simulink model "sysgenStreamedFFT"  (Simulink 7.4)
settings: Solver=VariableStepDiscrete  StartTime=0.0  StopTime=3000  RelTol=1e-3
values from neighbouring files (symbols this model uses):
  blue = blue(1:(min_x*min_y))    [makematrix.m]    (also in rgb.mat = [0 0 0 255 255 255 255 255 255 0 0 0 ... (256 elements, 256x)
  c = c(:)    [cellpipe_r13.m]    (also in cordic_sincos_script.m = xSignal; get_pipestr_r13.m = cellpipe_r13(pipestr))
  comp = [zeros(70,2) [zeros(2,66); comp; zeros(2,66)] zeros(70,2)]    [sysgenDWT_StopFcn.m]
undefined symbols (not defined in the file or in its folder): gcbh, xlBlockLoadCallback, xlipgetpartsetting
libraries: xbsIndex_r4 x117, dspxfrm3 x2, xbsCopyrightNotice_r4 x1
(part 2 of 3)

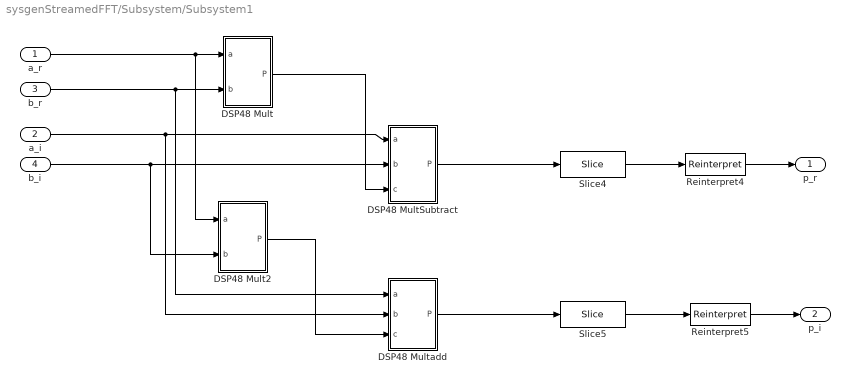
== system sysgenStreamedFFT/Subsystem/Subsystem1 ==
  a_r : Inport  OutDataType=sfix(16)  OutScaling=2^0
  a_i : Inport  Port=2  OutDataType=sfix(16)  OutScaling=2^0
  b_r : Inport  Port=3  OutDataType=sfix(16)  OutScaling=2^0
  b_i : Inport  Port=4  OutDataType=sfix(16)  OutScaling=2^0
  DSP48 Mult : Subsystem  LoadFcn=xlBlockLoadCallback(gcbh);  mask(Xilinx DSP48 Macro Block){infoedit=Macro function to simplify use of the DSP48 primitive, especially as a dynamic operator, portalist=a, portblist=b, portclist=, instrlist=|, pipeline_sgadvanced=, pipeline=Custom, pipeachoices_sgadvanced=, pipeachoices=1, pipebchoices_sgadvanced=, pipebchoices=1, pipecchoices_sgadvanced=, pipecchoices=off, pipepchoices_sgadvanced=, pipepchoices=on, pipemchoices_sgadvanced=, pipemchoices=on, pipectrlchoices_sgadvanced=, pipectrlchoices=on, pipemuxachoices_sgadvanced=, pipemuxachoices=0, pipemuxbchoices_sgadvanced=, pipemuxbchoices=0, pipemuxcchoices_sgadvanced=, pipemuxcchoices=0, pipemuxctrlchoices_sgadvanced=, pipemuxctrlchoices=0, pipeline_array_flag_sgadvanced=, pipeline_array_flag=off, custom_pipeline_cache=[1  1  0  1  1  1  0  0  0  0], precision_sgadvanced=, precision=Full, arith_type_sgadvanced=, arith_type=Signed  (2's comp), n_bits=12, bin_pt=12, bcout_sgadvanced=, bcout=off, acout_sgadvanced=, acout=off, carryout_sgadvanced=, carryout=off, carrycascout_sgadvanced=, carrycascout=off, pcout_sgadvanced=, pcout=off, rst_all_sgadvanced=, rst_all=off, rst_a_sgadvanced=, rst_a=off, rst_b_sgadvanced=, rst_b=off, rst_c_sgadvanced=, rst_c=off, rst_m_sgadvanced=, rst_m=off, rst_p_sgadvanced=, rst_p=off, rst_ctrl_sgadvanced=, rst_ctrl=off, ce_all_sgadvanced=, ce_all=off, ce_a_sgadvanced=, ce_a=off, ce_b_sgadvanced=, ce_b=off, ce_c_sgadvanced=, ce_c=off, ce_m_sgadvanced=, ce_m=off, ce_p_sgadvanced=, ce_p=off, ce_ctrl_sgadvanced=, ce_ctrl=off, dbl_ovrd_sgadvanced=, dbl_ovrd=off, synth_opt_sgadvanced=, synth_opt=on, errorlist=false, statestr=bf57e5972f25d56a71488d6ffddc6763, explicit_period=, period=1, maskdoc=, has_advanced_control=0, sggui_pos=200,234,478,593, block_type=dsp48macro, block_version=8.2.1, sg_icon_stat=45,67,2,1,white,blue,0,,right,, sg_mask_display=|, sg_list_contents=, sg_blockgui_xml=}
      mask instrlist=|
      | <html><head><meta name="qrichtext" content="1" /></head><body style="font-size:8pt;font-family:MS Shell Dlg">
      | <p>P=a*b</p>
      | </body></html>
      mask sg_mask_display=|
      | fprintf('','COMMENT: begin icon graphics');
      | patch([0 1 1 0 ],[0 0 1 1 ],[0.77 0.82 0.91]);
      | patch([0.222222 0.0666667 0.311111 0.0666667 0.222222 0.488889 0.555556 0.622222 0.911111 0.688889 0.466667 0.311111 0.555556 0.311111 0.466667 0.688889 0.911111 0.622222 0.555556 0.488889 0.222222 ],[0.238806 0.343284 0.507463 0.671642 0.776119 0.776119 0.731343 0.776119 0.776119 0.626866 0.776119 0.671642 0.507463 0.343284 0.238806 0.38806 0.238806 0.238806 0.283582 0.238806 0.238806 ],[0.98 0.96 0.92]);
      | plot([0 1 1 0 0 ],[0 0 1 1 0 ]);
      | fprintf('','COMMENT: end icon graphics');
      | fprintf('','COMMENT: begin icon text');
      | color('black');port_label('input',1,'a');
      | color('black');port_label('input',2,'b');
      | color('black');port_label('output',1,'P');
      | fprintf('','COMMENT: end icon text');
      mask prompts: infoedit ""; portalist "Inputs to port <tt>A</tt>"; portblist "Inputs to port <tt>B</tt>"; portclist "Inputs to port <tt>C</tt>"; instrlist "Instructions"; pipeline_sgadvanced ""; pipeline "Pipeline options"; pipeachoices_sgadvanced ""; pipeachoices "<tt>A</tt>"; pipebchoices_sgadvanced ""; pipebchoices "<tt>B</tt>"; pipecchoices_sgadvanced ""; pipecchoices "<tt>C</tt>"; pipepchoices_sgadvanced ""; pipepchoices "<tt>P</tt>"; pipemchoices_sgadvanced ""; pipemchoices "Multiplier"; pipectrlchoices_sgadvanced ""; pipectrlchoices "Controls (<tt>opmode</tt>, <tt>subtract</tt>,<br> <tt>carry_in</tt>, <tt>carry_in_sel</tt>)"; pipemuxachoices_sgadvanced ""; pipemuxachoices "MuxA"; pipemuxbchoices_sgadvanced ""; pipemuxbchoices "MuxB"; pipemuxcchoices_sgadvanced ""; pipemuxcchoices "MuxC"; pipemuxctrlchoices_sgadvanced ""; pipemuxctrlchoices "MuxCtrl"; pipeline_array_flag_sgadvanced ""; pipeline_array_flag "Define Using Array"; custom_pipeline_cache "Custom Pipeline Options([A,B,C,P,Ctrl,M,MuxA,MuxB,MuxC,MuxCtrl])"; precision_sgadvanced ""; arith_type_sgadvanced ""; arith_type "Output type"; n_bits "Number of bits"; bin_pt "Binary point"; bcout_sgadvanced ""; bcout "<tt>BCOUT</tt>"; acout_sgadvanced ""; acout "<tt>ACOUT</tt>"; carryout_sgadvanced ""; carryout "<tt>CARRYOUT</tt>"; carrycascout_sgadvanced ""; carrycascout "<tt>CARRYCASCOUT</tt>"; pcout_sgadvanced ""; pcout "<tt>PCOUT</tt>"; rst_all_sgadvanced ""; rst_all "<tt>Global Reset</tt>"; rst_a_sgadvanced ""; rst_a "Reset port for <tt>A</tt>"; rst_b_sgadvanced ""; rst_b "Reset port for <tt>B</tt>"; rst_c_sgadvanced ""; rst_c "Reset port for <tt>C</tt>"; rst_m_sgadvanced ""; rst_m "Reset port for multiplier"; rst_p_sgadvanced ""; rst_p "Reset port for <tt>P</tt>"; rst_ctrl_sgadvanced ""; rst_ctrl "Reset port for controls <br> (<tt>opmode</tt>, <tt>subtract</tt>,<br> <tt>carry_in</tt>, <tt>carry_in_sel</tt>)"; ce_all_sgadvanced ""; ce_all "<tt>Global Enable</tt>"; ce_a_sgadvanced ""; ce_a "Enable port for <tt>A</tt>"; ce_b_sgadvanced ""; ce_b "Enable port for <tt>B</tt>"; ce_c_sgadvanced ""; ce_c "Enable port for <tt>C</tt>"; ce_m_sgadvanced ""; ce_m "Enable port for multiplier"; ce_p_sgadvanced ""; ce_p "Enable port for <tt>P</tt>"; ce_ctrl_sgadvanced ""; ce_ctrl "Enable port for controls <br> (<tt>opmode</tt>, <tt>subtract</tt>,<br> <tt>carry_in</tt>, <tt>carry_in_sel</tt>)"; dbl_ovrd_sgadvanced ""; dbl_ovrd "Override with doubles"; synth_opt_sgadvanced ""; synth_opt "Use DSP48"; errorlist ""; statestr ""; explicit_period ""; period ""; maskdoc ""; has_advanced_control ""; sggui_pos ""; block_type ""; block_version ""; sg_icon_stat ""; sg_mask_display ""; sg_list_contents ""; sg_blockgui_xml ""
      mask help: Macro function to simplify use of the DSP48 primitive, especially as a dynamic operator
      mask init:
      | try
      |   tmp_gcb = gcb;
      |   tmp_gcbh = gcbh;
      |   xlMungeMaskParams;
      |   serialized_declarations = '{}';
      |   xldsp48macro_init();
      |   ptable_ = xlblockprep(get_param(tmp_gcb, 'MaskWSVariables'));
      | catch
      |   global dbgsysgen;
      |   if(~isempty(dbgsysgen) && dbgsysgen)
      |     e = regexprep(lasterr, '\n', '\nError: ');
      |     disp(['Error: While running MaskInit code on block ' tmp_gcb ': ' e]);
      |     error(e);
      |   end
      | end
      settings: CopyFcn=tmp_gcbh = gcbh;set_param(tmp_gcbh,'linkstatus','none');xlBlockMoveCallback(gcbh);  DeleteFcn=xlDestroyGui(gcbh);  ModelCloseFcn=xlDestroyGui(gcbh);  PreSaveFcn=xlBlockPreSaveCallback(gcbh);  PostSaveFcn=xlBlockPostSaveCallback(gcbh);  DestroyFcn=xlDestroyGui(gcbh);  OpenFcn=xlOpenGui(gcbh, 'dsp48macro_gui.xml', @dsp48macroenablement, @dsp48macroaction)  CloseFcn=xlDestroyGui(gcbh);  MoveFcn=xlBlockMoveCallback(gcbh);
      mask Help: xlWeb(xlhtmldoclink('DSP48 Macro'));
      mask StyleString: edit,edit,edit,edit,edit,edit,popup(External Registers|No External Registers|Custom),edit,popup(0|1|2),edit,popup(0|1|2),edit,checkbox,edit,checkbox,edit,checkbox,edit,checkbox,edit,popup(0|1|2),edit,popup(0|1|2),edit,popup(0|1|2),edit,popup(0|1|2),edit,checkbox,edit,edit,popup(Full|User Defined),edit,popup(Signed  (2's comp)|Unsigned),edit,edit,edit,checkbox,edit,checkbox,edit,checkbox,edit,checkbox,edit,checkbox,edit,checkbox,edit,checkbox,edit,checkbox,edit,checkbox,edit,checkbox,edit,checkbox,edit,checkbox,edit,checkbox,edit,checkbox,edit,checkbox,edit,checkbox,edit,checkbox,edit,checkbox,edit,checkbox,edit,checkbox,edit,checkbox,edit,edit,edit,edit,edit,edit,edit,edit,edit,edit,edit,edit,edit
      mask Display:
      | fprintf('','COMMENT: begin icon graphics');
      | patch([0 1 1 0 ],[0 0 1 1 ],[0.77 0.82 0.91]);
      | patch([0.222222 0.0666667 0.311111 0.0666667 0.222222 0.488889 0.555556 0.622222 0.911111 0.688889 0.466667 0.311111 0.555556 0.311111 0.466667 0.688889 0.911111 0.622222 0.555556 0.488889 0.222222 ],[0.238806 0.343284 0.507463 0.671642 0.776119 0.776119 0.731343 0.776119 0.776119 0.626866 0.776119 0.671642 0.507463 0.343284 0.238806 0.38806 0.238806 0.238806 0.283582 0.238806 0.238806 ],[0.98 0.96 0.92]);
      | plot([0 1 1 0 0 ],[0 0 1 1 0 ]);
      | fprintf('','COMMENT: end icon graphics');
      | fprintf('','COMMENT: begin icon text');
      | color('black');port_label('input',1,'a');
      | color('black');port_label('input',2,'b');
      | color('black');port_label('output',1,'P');
      | fprintf('','COMMENT: end icon text');
  DSP48 Mult2 : Subsystem  LoadFcn=xlBlockLoadCallback(gcbh);  mask(Xilinx DSP48 Macro Block){infoedit=Macro function to simplify use of the DSP48 primitive, especially as a dynamic operator, portalist=a, portblist=b, portclist=, instrlist=|, pipeline_sgadvanced=, pipeline=Custom, pipeachoices_sgadvanced=, pipeachoices=1, pipebchoices_sgadvanced=, pipebchoices=1, pipecchoices_sgadvanced=, pipecchoices=off, pipepchoices_sgadvanced=, pipepchoices=on, pipemchoices_sgadvanced=, pipemchoices=on, pipectrlchoices_sgadvanced=, pipectrlchoices=on, pipemuxachoices_sgadvanced=, pipemuxachoices=0, pipemuxbchoices_sgadvanced=, pipemuxbchoices=0, pipemuxcchoices_sgadvanced=, pipemuxcchoices=0, pipemuxctrlchoices_sgadvanced=, pipemuxctrlchoices=0, pipeline_array_flag_sgadvanced=, pipeline_array_flag=off, custom_pipeline_cache=[1  1  0  1  1  1  0  0  0  0], precision_sgadvanced=, precision=Full, arith_type_sgadvanced=, arith_type=Signed  (2's comp), n_bits=12, bin_pt=12, bcout_sgadvanced=, bcout=off, acout_sgadvanced=, acout=off, carryout_sgadvanced=, carryout=off, carrycascout_sgadvanced=, carrycascout=off, pcout_sgadvanced=, pcout=off, rst_all_sgadvanced=, rst_all=off, rst_a_sgadvanced=, rst_a=off, rst_b_sgadvanced=, rst_b=off, rst_c_sgadvanced=, rst_c=off, rst_m_sgadvanced=, rst_m=off, rst_p_sgadvanced=, rst_p=off, rst_ctrl_sgadvanced=, rst_ctrl=off, ce_all_sgadvanced=, ce_all=off, ce_a_sgadvanced=, ce_a=off, ce_b_sgadvanced=, ce_b=off, ce_c_sgadvanced=, ce_c=off, ce_m_sgadvanced=, ce_m=off, ce_p_sgadvanced=, ce_p=off, ce_ctrl_sgadvanced=, ce_ctrl=off, dbl_ovrd_sgadvanced=, dbl_ovrd=off, synth_opt_sgadvanced=, synth_opt=on, errorlist=false, statestr=bf57e5972f25d56a71488d6ffddc6763, explicit_period=, period=1, maskdoc=, has_advanced_control=0, sggui_pos=429,230,426,499, block_type=dsp48macro, block_version=8.2.1, sg_icon_stat=45,67,2,1,white,blue,0,,right,, sg_mask_display=|, sg_list_contents=, sg_blockgui_xml=}
      mask instrlist=|
      | <html><head><meta name="qrichtext" content="1" /></head><body style="font-size:8pt;font-family:MS Shell Dlg">
      | <p>P=a*b</p>
      | </body></html>
      mask sg_mask_display=|
      | fprintf('','COMMENT: begin icon graphics');
      | patch([0 1 1 0 ],[0 0 1 1 ],[0.77 0.82 0.91]);
      | patch([0.222222 0.0666667 0.311111 0.0666667 0.222222 0.488889 0.555556 0.622222 0.911111 0.688889 0.466667 0.311111 0.555556 0.311111 0.466667 0.688889 0.911111 0.622222 0.555556 0.488889 0.222222 ],[0.238806 0.343284 0.507463 0.671642 0.776119 0.776119 0.731343 0.776119 0.776119 0.626866 0.776119 0.671642 0.507463 0.343284 0.238806 0.38806 0.238806 0.238806 0.283582 0.238806 0.238806 ],[0.98 0.96 0.92]);
      | plot([0 1 1 0 0 ],[0 0 1 1 0 ]);
      | fprintf('','COMMENT: end icon graphics');
      | fprintf('','COMMENT: begin icon text');
      | color('black');port_label('input',1,'a');
      | color('black');port_label('input',2,'b');
      | color('black');port_label('output',1,'P');
      | fprintf('','COMMENT: end icon text');
      mask prompts: infoedit ""; portalist "Inputs to port <tt>A</tt>"; portblist "Inputs to port <tt>B</tt>"; portclist "Inputs to port <tt>C</tt>"; instrlist "Instructions"; pipeline_sgadvanced ""; pipeline "Pipeline options"; pipeachoices_sgadvanced ""; pipeachoices "<tt>A</tt>"; pipebchoices_sgadvanced ""; pipebchoices "<tt>B</tt>"; pipecchoices_sgadvanced ""; pipecchoices "<tt>C</tt>"; pipepchoices_sgadvanced ""; pipepchoices "<tt>P</tt>"; pipemchoices_sgadvanced ""; pipemchoices "Multiplier"; pipectrlchoices_sgadvanced ""; pipectrlchoices "Controls (<tt>opmode</tt>, <tt>subtract</tt>,<br> <tt>carry_in</tt>, <tt>carry_in_sel</tt>)"; pipemuxachoices_sgadvanced ""; pipemuxachoices "MuxA"; pipemuxbchoices_sgadvanced ""; pipemuxbchoices "MuxB"; pipemuxcchoices_sgadvanced ""; pipemuxcchoices "MuxC"; pipemuxctrlchoices_sgadvanced ""; pipemuxctrlchoices "MuxCtrl"; pipeline_array_flag_sgadvanced ""; pipeline_array_flag "Define Using Array"; custom_pipeline_cache "Custom Pipeline Options([A,B,C,P,Ctrl,M,MuxA,MuxB,MuxC,MuxCtrl])"; precision_sgadvanced ""; arith_type_sgadvanced ""; arith_type "Output type"; n_bits "Number of bits"; bin_pt "Binary point"; bcout_sgadvanced ""; bcout "<tt>BCOUT</tt>"; acout_sgadvanced ""; acout "<tt>ACOUT</tt>"; carryout_sgadvanced ""; carryout "<tt>CARRYOUT</tt>"; carrycascout_sgadvanced ""; carrycascout "<tt>CARRYCASCOUT</tt>"; pcout_sgadvanced ""; pcout "<tt>PCOUT</tt>"; rst_all_sgadvanced ""; rst_all "<tt>Global Reset</tt>"; rst_a_sgadvanced ""; rst_a "Reset port for <tt>A</tt>"; rst_b_sgadvanced ""; rst_b "Reset port for <tt>B</tt>"; rst_c_sgadvanced ""; rst_c "Reset port for <tt>C</tt>"; rst_m_sgadvanced ""; rst_m "Reset port for multiplier"; rst_p_sgadvanced ""; rst_p "Reset port for <tt>P</tt>"; rst_ctrl_sgadvanced ""; rst_ctrl "Reset port for controls <br> (<tt>opmode</tt>, <tt>subtract</tt>,<br> <tt>carry_in</tt>, <tt>carry_in_sel</tt>)"; ce_all_sgadvanced ""; ce_all "<tt>Global Enable</tt>"; ce_a_sgadvanced ""; ce_a "Enable port for <tt>A</tt>"; ce_b_sgadvanced ""; ce_b "Enable port for <tt>B</tt>"; ce_c_sgadvanced ""; ce_c "Enable port for <tt>C</tt>"; ce_m_sgadvanced ""; ce_m "Enable port for multiplier"; ce_p_sgadvanced ""; ce_p "Enable port for <tt>P</tt>"; ce_ctrl_sgadvanced ""; ce_ctrl "Enable port for controls <br> (<tt>opmode</tt>, <tt>subtract</tt>,<br> <tt>carry_in</tt>, <tt>carry_in_sel</tt>)"; dbl_ovrd_sgadvanced ""; dbl_ovrd "Override with doubles"; synth_opt_sgadvanced ""; synth_opt "Use DSP48"; errorlist ""; statestr ""; explicit_period ""; period ""; maskdoc ""; has_advanced_control ""; sggui_pos ""; block_type ""; block_version ""; sg_icon_stat ""; sg_mask_display ""; sg_list_contents ""; sg_blockgui_xml ""
      mask help: Macro function to simplify use of the DSP48 primitive, especially as a dynamic operator
      mask init: same as sysgenStreamedFFT/Subsystem/Subsystem1/DSP48 Mult
      settings: CopyFcn=tmp_gcbh = gcbh;set_param(tmp_gcbh,'linkstatus','none');xlBlockMoveCallback(gcbh);  DeleteFcn=xlDestroyGui(gcbh);  ModelCloseFcn=xlDestroyGui(gcbh);  PreSaveFcn=xlBlockPreSaveCallback(gcbh);  PostSaveFcn=xlBlockPostSaveCallback(gcbh);  DestroyFcn=xlDestroyGui(gcbh);  OpenFcn=xlOpenGui(gcbh, 'dsp48macro_gui.xml', @dsp48macroenablement, @dsp48macroaction)  CloseFcn=xlDestroyGui(gcbh);  MoveFcn=xlBlockMoveCallback(gcbh);
      mask Help: xlWeb(xlhtmldoclink('DSP48 Macro'));
      mask StyleString: edit,edit,edit,edit,edit,edit,popup(External Registers|No External Registers|Custom),edit,popup(0|1|2),edit,popup(0|1|2),edit,checkbox,edit,checkbox,edit,checkbox,edit,checkbox,edit,popup(0|1|2),edit,popup(0|1|2),edit,popup(0|1|2),edit,popup(0|1|2),edit,checkbox,edit,edit,popup(Full|User Defined),edit,popup(Signed  (2's comp)|Unsigned),edit,edit,edit,checkbox,edit,checkbox,edit,checkbox,edit,checkbox,edit,checkbox,edit,checkbox,edit,checkbox,edit,checkbox,edit,checkbox,edit,checkbox,edit,checkbox,edit,checkbox,edit,checkbox,edit,checkbox,edit,checkbox,edit,checkbox,edit,checkbox,edit,checkbox,edit,checkbox,edit,checkbox,edit,checkbox,edit,edit,edit,edit,edit,edit,edit,edit,edit,edit,edit,edit,edit
      mask Display:
      | fprintf('','COMMENT: begin icon graphics');
      | patch([0 1 1 0 ],[0 0 1 1 ],[0.77 0.82 0.91]);
      | patch([0.222222 0.0666667 0.311111 0.0666667 0.222222 0.488889 0.555556 0.622222 0.911111 0.688889 0.466667 0.311111 0.555556 0.311111 0.466667 0.688889 0.911111 0.622222 0.555556 0.488889 0.222222 ],[0.238806 0.343284 0.507463 0.671642 0.776119 0.776119 0.731343 0.776119 0.776119 0.626866 0.776119 0.671642 0.507463 0.343284 0.238806 0.38806 0.238806 0.238806 0.283582 0.238806 0.238806 ],[0.98 0.96 0.92]);
      | plot([0 1 1 0 0 ],[0 0 1 1 0 ]);
      | fprintf('','COMMENT: end icon graphics');
      | fprintf('','COMMENT: begin icon text');
      | color('black');port_label('input',1,'a');
      | color('black');port_label('input',2,'b');
      | color('black');port_label('output',1,'P');
      | fprintf('','COMMENT: end icon text');
  DSP48 MultSubtract : Subsystem  LoadFcn=xlBlockLoadCallback(gcbh);  mask(Xilinx DSP48 Macro Block){infoedit=Macro function to simplify use of the DSP48 primitive, especially as a dynamic operator, portalist=a, portblist=b, portclist=c, instrlist=|, pipeline_sgadvanced=, pipeline=Custom, pipeachoices_sgadvanced=, pipeachoices=1, pipebchoices_sgadvanced=, pipebchoices=1, pipecchoices_sgadvanced=, pipecchoices=on, pipepchoices_sgadvanced=, pipepchoices=on, pipemchoices_sgadvanced=, pipemchoices=on, pipectrlchoices_sgadvanced=, pipectrlchoices=on, pipemuxachoices_sgadvanced=, pipemuxachoices=0, pipemuxbchoices_sgadvanced=, pipemuxbchoices=0, pipemuxcchoices_sgadvanced=, pipemuxcchoices=0, pipemuxctrlchoices_sgadvanced=, pipemuxctrlchoices=0, pipeline_array_flag_sgadvanced=, pipeline_array_flag=off, custom_pipeline_cache=[1  1  1  1  1  1  0  0  0  0], precision_sgadvanced=, precision=Full, arith_type_sgadvanced=, arith_type=Signed  (2's comp), n_bits=12, bin_pt=12, bcout_sgadvanced=, bcout=off, acout_sgadvanced=, acout=off, carryout_sgadvanced=, carryout=off, carrycascout_sgadvanced=, carrycascout=off, pcout_sgadvanced=, pcout=off, rst_all_sgadvanced=, rst_all=off, rst_a_sgadvanced=, rst_a=off, rst_b_sgadvanced=, rst_b=off, rst_c_sgadvanced=, rst_c=off, rst_m_sgadvanced=, rst_m=off, rst_p_sgadvanced=, rst_p=off, rst_ctrl_sgadvanced=, rst_ctrl=off, ce_all_sgadvanced=, ce_all=off, ce_a_sgadvanced=, ce_a=off, ce_b_sgadvanced=, ce_b=off, ce_c_sgadvanced=, ce_c=off, ce_m_sgadvanced=, ce_m=off, ce_p_sgadvanced=, ce_p=off, ce_ctrl_sgadvanced=, ce_ctrl=off, dbl_ovrd_sgadvanced=, dbl_ovrd=off, synth_opt_sgadvanced=, synth_opt=on, errorlist=false, statestr=e43659f44466f7be952996a9572528ef, explicit_period=, period=1, maskdoc=, has_advanced_control=0, sggui_pos=429,230,478,550, block_type=dsp48macro, block_version=8.2.1, sg_icon_stat=45,74,3,1,white,blue,0,,right,, sg_mask_display=|, sg_list_contents=, sg_blockgui_xml=}
      mask instrlist=|
      | <html><head><meta name="qrichtext" content="1" /></head><body style="font-size:8pt;font-family:MS Shell Dlg">
      | <p>P=c-a*b</p>
      | </body></html>
      mask sg_mask_display=|
      | fprintf('','COMMENT: begin icon graphics');
      | patch([0 1 1 0 ],[0 0 1 1 ],[0.77 0.82 0.91]);
      | patch([0.222222 0.0666667 0.311111 0.0666667 0.222222 0.488889 0.555556 0.622222 0.911111 0.688889 0.466667 0.311111 0.555556 0.311111 0.466667 0.688889 0.911111 0.622222 0.555556 0.488889 0.222222 ],[0.256757 0.351351 0.5 0.648649 0.743243 0.743243 0.702703 0.743243 0.743243 0.608108 0.743243 0.648649 0.5 0.351351 0.256757 0.391892 0.256757 0.256757 0.297297 0.256757 0.256757 ],[0.98 0.96 0.92]);
      | plot([0 1 1 0 0 ],[0 0 1 1 0 ]);
      | fprintf('','COMMENT: end icon graphics');
      | fprintf('','COMMENT: begin icon text');
      | color('black');port_label('input',1,'a');
      | color('black');port_label('input',2,'b');
      | color('black');port_label('input',3,'c');
      | color('black');port_label('output',1,'P');
      | fprintf('','COMMENT: end icon text');
      mask prompts: infoedit ""; portalist "Inputs to port <tt>A</tt>"; portblist "Inputs to port <tt>B</tt>"; portclist "Inputs to port <tt>C</tt>"; instrlist "Instructions"; pipeline_sgadvanced ""; pipeline "Pipeline options"; pipeachoices_sgadvanced ""; pipeachoices "<tt>A</tt>"; pipebchoices_sgadvanced ""; pipebchoices "<tt>B</tt>"; pipecchoices_sgadvanced ""; pipecchoices "<tt>C</tt>"; pipepchoices_sgadvanced ""; pipepchoices "<tt>P</tt>"; pipemchoices_sgadvanced ""; pipemchoices "Multiplier"; pipectrlchoices_sgadvanced ""; pipectrlchoices "Controls (<tt>opmode</tt>, <tt>subtract</tt>,<br> <tt>carry_in</tt>, <tt>carry_in_sel</tt>)"; pipemuxachoices_sgadvanced ""; pipemuxachoices "MuxA"; pipemuxbchoices_sgadvanced ""; pipemuxbchoices "MuxB"; pipemuxcchoices_sgadvanced ""; pipemuxcchoices "MuxC"; pipemuxctrlchoices_sgadvanced ""; pipemuxctrlchoices "MuxCtrl"; pipeline_array_flag_sgadvanced ""; pipeline_array_flag "Define Using Array"; custom_pipeline_cache "Custom Pipeline Options([A,B,C,P,Ctrl,M,MuxA,MuxB,MuxC,MuxCtrl])"; precision_sgadvanced ""; arith_type_sgadvanced ""; arith_type "Output type"; n_bits "Number of bits"; bin_pt "Binary point"; bcout_sgadvanced ""; bcout "<tt>BCOUT</tt>"; acout_sgadvanced ""; acout "<tt>ACOUT</tt>"; carryout_sgadvanced ""; carryout "<tt>CARRYOUT</tt>"; carrycascout_sgadvanced ""; carrycascout "<tt>CARRYCASCOUT</tt>"; pcout_sgadvanced ""; pcout "<tt>PCOUT</tt>"; rst_all_sgadvanced ""; rst_all "<tt>Global Reset</tt>"; rst_a_sgadvanced ""; rst_a "Reset port for <tt>A</tt>"; rst_b_sgadvanced ""; rst_b "Reset port for <tt>B</tt>"; rst_c_sgadvanced ""; rst_c "Reset port for <tt>C</tt>"; rst_m_sgadvanced ""; rst_m "Reset port for multiplier"; rst_p_sgadvanced ""; rst_p "Reset port for <tt>P</tt>"; rst_ctrl_sgadvanced ""; rst_ctrl "Reset port for controls <br> (<tt>opmode</tt>, <tt>subtract</tt>,<br> <tt>carry_in</tt>, <tt>carry_in_sel</tt>)"; ce_all_sgadvanced ""; ce_all "<tt>Global Enable</tt>"; ce_a_sgadvanced ""; ce_a "Enable port for <tt>A</tt>"; ce_b_sgadvanced ""; ce_b "Enable port for <tt>B</tt>"; ce_c_sgadvanced ""; ce_c "Enable port for <tt>C</tt>"; ce_m_sgadvanced ""; ce_m "Enable port for multiplier"; ce_p_sgadvanced ""; ce_p "Enable port for <tt>P</tt>"; ce_ctrl_sgadvanced ""; ce_ctrl "Enable port for controls <br> (<tt>opmode</tt>, <tt>subtract</tt>,<br> <tt>carry_in</tt>, <tt>carry_in_sel</tt>)"; dbl_ovrd_sgadvanced ""; dbl_ovrd "Override with doubles"; synth_opt_sgadvanced ""; synth_opt "Use DSP48"; errorlist ""; statestr ""; explicit_period ""; period ""; maskdoc ""; has_advanced_control ""; sggui_pos ""; block_type ""; block_version ""; sg_icon_stat ""; sg_mask_display ""; sg_list_contents ""; sg_blockgui_xml ""
      mask help: Macro function to simplify use of the DSP48 primitive, especially as a dynamic operator
      mask init: same as sysgenStreamedFFT/Subsystem/Subsystem1/DSP48 Mult
      settings: CopyFcn=tmp_gcbh = gcbh;set_param(tmp_gcbh,'linkstatus','none');xlBlockMoveCallback(gcbh);  DeleteFcn=xlDestroyGui(gcbh);  ModelCloseFcn=xlDestroyGui(gcbh);  PreSaveFcn=xlBlockPreSaveCallback(gcbh);  PostSaveFcn=xlBlockPostSaveCallback(gcbh);  DestroyFcn=xlDestroyGui(gcbh);  OpenFcn=xlOpenGui(gcbh, 'dsp48macro_gui.xml', @dsp48macroenablement, @dsp48macroaction)  CloseFcn=xlDestroyGui(gcbh);  MoveFcn=xlBlockMoveCallback(gcbh);
      mask Help: xlWeb(xlhtmldoclink('DSP48 Macro'));
      mask StyleString: edit,edit,edit,edit,edit,edit,popup(External Registers|No External Registers|Custom),edit,popup(0|1|2),edit,popup(0|1|2),edit,checkbox,edit,checkbox,edit,checkbox,edit,checkbox,edit,popup(0|1|2),edit,popup(0|1|2),edit,popup(0|1|2),edit,popup(0|1|2),edit,checkbox,edit,edit,popup(Full|User Defined),edit,popup(Signed  (2's comp)|Unsigned),edit,edit,edit,checkbox,edit,checkbox,edit,checkbox,edit,checkbox,edit,checkbox,edit,checkbox,edit,checkbox,edit,checkbox,edit,checkbox,edit,checkbox,edit,checkbox,edit,checkbox,edit,checkbox,edit,checkbox,edit,checkbox,edit,checkbox,edit,checkbox,edit,checkbox,edit,checkbox,edit,checkbox,edit,checkbox,edit,edit,edit,edit,edit,edit,edit,edit,edit,edit,edit,edit,edit
      mask Display:
      | fprintf('','COMMENT: begin icon graphics');
      | patch([0 1 1 0 ],[0 0 1 1 ],[0.77 0.82 0.91]);
      | patch([0.222222 0.0666667 0.311111 0.0666667 0.222222 0.488889 0.555556 0.622222 0.911111 0.688889 0.466667 0.311111 0.555556 0.311111 0.466667 0.688889 0.911111 0.622222 0.555556 0.488889 0.222222 ],[0.256757 0.351351 0.5 0.648649 0.743243 0.743243 0.702703 0.743243 0.743243 0.608108 0.743243 0.648649 0.5 0.351351 0.256757 0.391892 0.256757 0.256757 0.297297 0.256757 0.256757 ],[0.98 0.96 0.92]);
      | plot([0 1 1 0 0 ],[0 0 1 1 0 ]);
      | fprintf('','COMMENT: end icon graphics');
      | fprintf('','COMMENT: begin icon text');
      | color('black');port_label('input',1,'a');
      | color('black');port_label('input',2,'b');
      | color('black');port_label('input',3,'c');
      | color('black');port_label('output',1,'P');
      | fprintf('','COMMENT: end icon text');
  DSP48 Multadd : Subsystem  LoadFcn=xlBlockLoadCallback(gcbh);  mask(Xilinx DSP48 Macro Block){infoedit=Macro function to simplify use of the DSP48 primitive, especially as a dynamic operator, portalist=a, portblist=b, portclist=c, instrlist=|, pipeline_sgadvanced=, pipeline=Custom, pipeachoices_sgadvanced=, pipeachoices=1, pipebchoices_sgadvanced=, pipebchoices=1, pipecchoices_sgadvanced=, pipecchoices=on, pipepchoices_sgadvanced=, pipepchoices=on, pipemchoices_sgadvanced=, pipemchoices=on, pipectrlchoices_sgadvanced=, pipectrlchoices=on, pipemuxachoices_sgadvanced=, pipemuxachoices=0, pipemuxbchoices_sgadvanced=, pipemuxbchoices=0, pipemuxcchoices_sgadvanced=, pipemuxcchoices=0, pipemuxctrlchoices_sgadvanced=, pipemuxctrlchoices=0, pipeline_array_flag_sgadvanced=, pipeline_array_flag=off, custom_pipeline_cache=[1  1  1  1  1  1  0  0  0  0], precision_sgadvanced=, precision=Full, arith_type_sgadvanced=, arith_type=Signed  (2's comp), n_bits=12, bin_pt=12, bcout_sgadvanced=, bcout=off, acout_sgadvanced=, acout=off, carryout_sgadvanced=, carryout=off, carrycascout_sgadvanced=, carrycascout=off, pcout_sgadvanced=, pcout=off, rst_all_sgadvanced=, rst_all=off, rst_a_sgadvanced=, rst_a=off, rst_b_sgadvanced=, rst_b=off, rst_c_sgadvanced=, rst_c=off, rst_m_sgadvanced=, rst_m=off, rst_p_sgadvanced=, rst_p=off, rst_ctrl_sgadvanced=, rst_ctrl=off, ce_all_sgadvanced=, ce_all=off, ce_a_sgadvanced=, ce_a=off, ce_b_sgadvanced=, ce_b=off, ce_c_sgadvanced=, ce_c=off, ce_m_sgadvanced=, ce_m=off, ce_p_sgadvanced=, ce_p=off, ce_ctrl_sgadvanced=, ce_ctrl=off, dbl_ovrd_sgadvanced=, dbl_ovrd=off, synth_opt_sgadvanced=, synth_opt=on, errorlist=false, statestr=e63290abb6eb2d1c13234b0ccbf6f8a4, explicit_period=, period=1, maskdoc=, has_advanced_control=0, sggui_pos=429,230,426,499, block_type=dsp48macro, block_version=8.2.1, sg_icon_stat=45,68,3,1,white,blue,0,,right,, sg_mask_display=|, sg_list_contents=, sg_blockgui_xml=}
      mask instrlist=|
      | <html><head><meta name="qrichtext" content="1" /></head><body style="font-size:8pt;font-family:MS Shell Dlg">
      | <p>P=c+a*b</p>
      | </body></html>
      mask sg_mask_display=|
      | fprintf('','COMMENT: begin icon graphics');
      | patch([0 1 1 0 ],[0 0 1 1 ],[0.77 0.82 0.91]);
      | patch([0.222222 0.0666667 0.311111 0.0666667 0.222222 0.488889 0.555556 0.622222 0.911111 0.688889 0.466667 0.311111 0.555556 0.311111 0.466667 0.688889 0.911111 0.622222 0.555556 0.488889 0.222222 ],[0.235294 0.338235 0.5 0.661765 0.764706 0.764706 0.720588 0.764706 0.764706 0.617647 0.764706 0.661765 0.5 0.338235 0.235294 0.382353 0.235294 0.235294 0.279412 0.235294 0.235294 ],[0.98 0.96 0.92]);
      | plot([0 1 1 0 0 ],[0 0 1 1 0 ]);
      | fprintf('','COMMENT: end icon graphics');
      | fprintf('','COMMENT: begin icon text');
      | color('black');port_label('input',1,'a');
      | color('black');port_label('input',2,'b');
      | color('black');port_label('input',3,'c');
      | color('black');port_label('output',1,'P');
      | fprintf('','COMMENT: end icon text');
      mask prompts: infoedit ""; portalist "Inputs to port <tt>A</tt>"; portblist "Inputs to port <tt>B</tt>"; portclist "Inputs to port <tt>C</tt>"; instrlist "Instructions"; pipeline_sgadvanced ""; pipeline "Pipeline options"; pipeachoices_sgadvanced ""; pipeachoices "<tt>A</tt>"; pipebchoices_sgadvanced ""; pipebchoices "<tt>B</tt>"; pipecchoices_sgadvanced ""; pipecchoices "<tt>C</tt>"; pipepchoices_sgadvanced ""; pipepchoices "<tt>P</tt>"; pipemchoices_sgadvanced ""; pipemchoices "Multiplier"; pipectrlchoices_sgadvanced ""; pipectrlchoices "Controls (<tt>opmode</tt>, <tt>subtract</tt>,<br> <tt>carry_in</tt>, <tt>carry_in_sel</tt>)"; pipemuxachoices_sgadvanced ""; pipemuxachoices "MuxA"; pipemuxbchoices_sgadvanced ""; pipemuxbchoices "MuxB"; pipemuxcchoices_sgadvanced ""; pipemuxcchoices "MuxC"; pipemuxctrlchoices_sgadvanced ""; pipemuxctrlchoices "MuxCtrl"; pipeline_array_flag_sgadvanced ""; pipeline_array_flag "Define Using Array"; custom_pipeline_cache "Custom Pipeline Options([A,B,C,P,Ctrl,M,MuxA,MuxB,MuxC,MuxCtrl])"; precision_sgadvanced ""; arith_type_sgadvanced ""; arith_type "Output type"; n_bits "Number of bits"; bin_pt "Binary point"; bcout_sgadvanced ""; bcout "<tt>BCOUT</tt>"; acout_sgadvanced ""; acout "<tt>ACOUT</tt>"; carryout_sgadvanced ""; carryout "<tt>CARRYOUT</tt>"; carrycascout_sgadvanced ""; carrycascout "<tt>CARRYCASCOUT</tt>"; pcout_sgadvanced ""; pcout "<tt>PCOUT</tt>"; rst_all_sgadvanced ""; rst_all "<tt>Global Reset</tt>"; rst_a_sgadvanced ""; rst_a "Reset port for <tt>A</tt>"; rst_b_sgadvanced ""; rst_b "Reset port for <tt>B</tt>"; rst_c_sgadvanced ""; rst_c "Reset port for <tt>C</tt>"; rst_m_sgadvanced ""; rst_m "Reset port for multiplier"; rst_p_sgadvanced ""; rst_p "Reset port for <tt>P</tt>"; rst_ctrl_sgadvanced ""; rst_ctrl "Reset port for controls <br> (<tt>opmode</tt>, <tt>subtract</tt>,<br> <tt>carry_in</tt>, <tt>carry_in_sel</tt>)"; ce_all_sgadvanced ""; ce_all "<tt>Global Enable</tt>"; ce_a_sgadvanced ""; ce_a "Enable port for <tt>A</tt>"; ce_b_sgadvanced ""; ce_b "Enable port for <tt>B</tt>"; ce_c_sgadvanced ""; ce_c "Enable port for <tt>C</tt>"; ce_m_sgadvanced ""; ce_m "Enable port for multiplier"; ce_p_sgadvanced ""; ce_p "Enable port for <tt>P</tt>"; ce_ctrl_sgadvanced ""; ce_ctrl "Enable port for controls <br> (<tt>opmode</tt>, <tt>subtract</tt>,<br> <tt>carry_in</tt>, <tt>carry_in_sel</tt>)"; dbl_ovrd_sgadvanced ""; dbl_ovrd "Override with doubles"; synth_opt_sgadvanced ""; synth_opt "Use DSP48"; errorlist ""; statestr ""; explicit_period ""; period ""; maskdoc ""; has_advanced_control ""; sggui_pos ""; block_type ""; block_version ""; sg_icon_stat ""; sg_mask_display ""; sg_list_contents ""; sg_blockgui_xml ""
      mask help: Macro function to simplify use of the DSP48 primitive, especially as a dynamic operator
      mask init: same as sysgenStreamedFFT/Subsystem/Subsystem1/DSP48 Mult
      settings: CopyFcn=tmp_gcbh = gcbh;set_param(tmp_gcbh,'linkstatus','none');xlBlockMoveCallback(gcbh);  DeleteFcn=xlDestroyGui(gcbh);  ModelCloseFcn=xlDestroyGui(gcbh);  PreSaveFcn=xlBlockPreSaveCallback(gcbh);  PostSaveFcn=xlBlockPostSaveCallback(gcbh);  DestroyFcn=xlDestroyGui(gcbh);  OpenFcn=xlOpenGui(gcbh, 'dsp48macro_gui.xml', @dsp48macroenablement, @dsp48macroaction)  CloseFcn=xlDestroyGui(gcbh);  MoveFcn=xlBlockMoveCallback(gcbh);
      mask Help: xlWeb(xlhtmldoclink('DSP48 Macro'));
      mask StyleString: edit,edit,edit,edit,edit,edit,popup(External Registers|No External Registers|Custom),edit,popup(0|1|2),edit,popup(0|1|2),edit,checkbox,edit,checkbox,edit,checkbox,edit,checkbox,edit,popup(0|1|2),edit,popup(0|1|2),edit,popup(0|1|2),edit,popup(0|1|2),edit,checkbox,edit,edit,popup(Full|User Defined),edit,popup(Signed  (2's comp)|Unsigned),edit,edit,edit,checkbox,edit,checkbox,edit,checkbox,edit,checkbox,edit,checkbox,edit,checkbox,edit,checkbox,edit,checkbox,edit,checkbox,edit,checkbox,edit,checkbox,edit,checkbox,edit,checkbox,edit,checkbox,edit,checkbox,edit,checkbox,edit,checkbox,edit,checkbox,edit,checkbox,edit,checkbox,edit,checkbox,edit,edit,edit,edit,edit,edit,edit,edit,edit,edit,edit,edit,edit
      mask Display:
      | fprintf('','COMMENT: begin icon graphics');
      | patch([0 1 1 0 ],[0 0 1 1 ],[0.77 0.82 0.91]);
      | patch([0.222222 0.0666667 0.311111 0.0666667 0.222222 0.488889 0.555556 0.622222 0.911111 0.688889 0.466667 0.311111 0.555556 0.311111 0.466667 0.688889 0.911111 0.622222 0.555556 0.488889 0.222222 ],[0.235294 0.338235 0.5 0.661765 0.764706 0.764706 0.720588 0.764706 0.764706 0.617647 0.764706 0.661765 0.5 0.338235 0.235294 0.382353 0.235294 0.235294 0.279412 0.235294 0.235294 ],[0.98 0.96 0.92]);
      | plot([0 1 1 0 0 ],[0 0 1 1 0 ]);
      | fprintf('','COMMENT: end icon graphics');
      | fprintf('','COMMENT: begin icon text');
      | color('black');port_label('input',1,'a');
      | color('black');port_label('input',2,'b');
      | color('black');port_label('input',3,'c');
      | color('black');port_label('output',1,'P');
      | fprintf('','COMMENT: end icon text');
  Reinterpret4 : xbsIndex_r4/Reinterpret  force_arith_type=on  arith_type="Signed  (2's comp)"  force_bin_pt=on  bin_pt=12  block_type=reinterpret
      settings: infoedit="Changes signal type without altering the binary representation.   You can changed the signal between signed and unsigned, and relocate the binary point.<P><P>Hardware notes: In hardware this block costs nothing.<P><P>Example:  Suppose the input is 6 bits wide, signed, with 2 fractional bits, and the output is forced to unsigned with 0 fractional bits.  Then an input of -2.0 (1110.00 in binary 2's complement) becomes an output of 56 (111000 in binary)."  block_version=9.1
  Reinterpret5 : xbsIndex_r4/Reinterpret  force_arith_type=on  arith_type="Signed  (2's comp)"  force_bin_pt=on  bin_pt=12  block_type=reinterpret
      settings: infoedit="Changes signal type without altering the binary representation.   You can changed the signal between signed and unsigned, and relocate the binary point.<P><P>Hardware notes: In hardware this block costs nothing.<P><P>Example:  Suppose the input is 6 bits wide, signed, with 2 fractional bits, and the output is forced to unsigned with 0 fractional bits.  Then an input of -2.0 (1110.00 in binary 2's complement) becomes an output of 56 (111000 in binary)."  block_version=9.1
  Slice4 : xbsIndex_r4/Slice  nbits=13  boolean_output=off  mode=Lower Bit Location + Width  bit1=0  base1=MSB of Input  bit0=0  base0=LSB of Input  dbl_ovrd=off  block_type=slice
      settings: infoedit="Extracts a given range of bits from each input sample and presents it at the output.  The output type is ordinarily unsigned with binary point at zero, but can be Boolean when the slice is one bit wide.<P><P>Hardware notes: In hardware this block costs nothing."  block_version=9.1
  Slice5 : xbsIndex_r4/Slice  nbits=13  boolean_output=off  mode=Lower Bit Location + Width  bit1=0  base1=MSB of Input  bit0=0  base0=LSB of Input  dbl_ovrd=off  block_type=slice
      settings: infoedit="Extracts a given range of bits from each input sample and presents it at the output.  The output type is ordinarily unsigned with binary point at zero, but can be Boolean when the slice is one bit wide.<P><P>Hardware notes: In hardware this block costs nothing."  block_version=9.1
  p_r : Outport  OutDataType=sfix(16)  OutScaling=2^0
  p_i : Outport  Port=2  OutDataType=sfix(16)  OutScaling=2^0
  wires:
  DSP48 Multadd/1(P) -> Slice5/1
  DSP48 MultSubtract/1(P) -> Slice4/1
  a_r/1 -> DSP48 Mult/1(a), DSP48 Mult2/1(a)
  b_i/1 -> DSP48 MultSubtract/2(b), DSP48 Mult2/2(b)
  b_r/1 -> DSP48 Mult/2(b), DSP48 Multadd/1(a)
  a_i/1 -> DSP48 MultSubtract/1(a), DSP48 Multadd/2(b)
  Slice4/1 -> Reinterpret4/1
  Slice5/1 -> Reinterpret5/1
  Reinterpret4/1 -> p_r/1
  Reinterpret5/1 -> p_i/1
  DSP48 Mult/1(P) -> DSP48 MultSubtract/3(c)
  DSP48 Mult2/1(P) -> DSP48 Multadd/3(c)

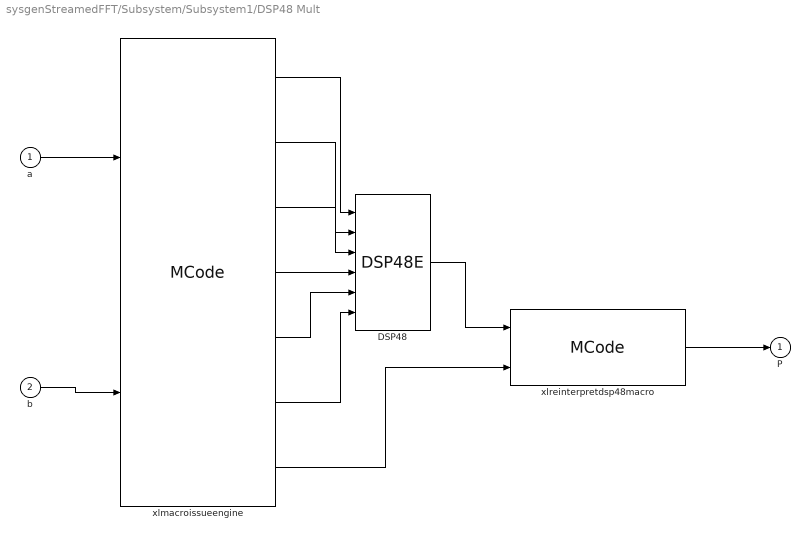
== system sysgenStreamedFFT/Subsystem/Subsystem1/DSP48 Mult ==
  a : Inport  OutDataType=sfix(16)  OutScaling=2^0
  b : Inport  Port=2  OutDataType=sfix(16)  OutScaling=2^0
  DSP48 : xbsIndex_r4/DSP48E  use_a=Direct from A Port  use_b=Direct from B Port  pattern_from_creg=off  pattern='000000000000'  mask_from_creg=off  pattern_mask='000000000000'  reset_preg=off  sel_rounding_mask=Select mask  use_op=off  use_creg=off  rst_all=off  en_all=off  use_pcin=off  use_carrycascin=off  use_multsignin=off  use_carryout=off  use_patterndetect=off  use_patternbdetect=off  use_overflow=off  use_underflow=off  use_acout=off  use_bcout=off  use_pcout=off  use_multsignout=off  use_carrycascout=off  pipeline_a=1  pipeline_b=1  pipeline_acout=1  pipeline_bcout=1  pipeline_c=off  pipeline_p=on  pipeline_mult=on  pipeline_opmode=on  pipeline_alumode=on  pipeline_carryin=on  pipeline_carryinsel=on  rst_a=off  rst_b=off  rst_c=off  rst_mult=off  rst_p=off  rst_carry_in=off  rst_alumode=off  rst_ctrl=off  en_a1=off  en_a2=off  en_b1=off  en_b2=off  en_c=off  en_mult=off  en_p=off  en_carry_in=off  en_alumode=off  en_multcarryin=off  en_ctrl=off  use_synth_model=off  addsub_mode=ONE48  xl_useadderonly=off  block_type=dsp48e
      settings: block_version=11.3
  xlmacroissueengine : xbsIndex_r4/MCode  mfname=xlissue_engine_v5  explicit_period=off  period=inf  dbl_ovrd=off  enable_stdout=off  enable_debug=off  suppress_output=on  defparams={'id_a1', 0,'id_a2', 0,'id_a3', 0,'id_a4', 0,'id_a5', 0,'id_a6', 0,'id_a7', 0,'id_b1', 0,'id_b2', 0,'id_b3', 0,'id_b4', 0,'id_b5', 0,'id_b6', 0,'id_b7', 0,'id_c0', 0,'id_c1', 0,'id_c2', 0,'id_c3', 0,'id_c4', 0,'id_c5', 0,'id_c6', 0,'id_c7', 0,'op_const0',5,'op_const1', 0,'op_const2', 0,'op_const3', 0,'op_const4', 0,'op_const5', 0,'op_const6', 0,'op_const7', 0,'alumode_const0',0,'alumode_const1', 0,'alumode_const2', 0,'alumode_const3', 0,'alumode_const4', 0,'alumode_const5', 0,'alumode_const6', 0,'alumode_const7', 0,'carry_in_sel0',0,'carry_in_sel1', 0,'carry_in_sel2', 0,'carry_in_sel3', 0,'carry_in_sel4', 0,'carry_in_sel5', 0,'carry_in_sel6', 0,'carry_in_sel7', 0,'external_cin0', 0,'external_cin1', 0,'external_cin2', 0,'external_cin3', 0,'external_cin4', 0,'external_cin5', 0,'external_cin6', 0,'external_cin7', 0,'reg_a',0,'reg_b',0,'reg_c',0,'reg_op',0,'mode0', 1,'mode1', 0,'mode2', 0,'mode3', 0,'mode4', 0,'mode5', 0,'mode6', 0,'mode7', 0,'ce_all',true,'use_ce_all',false,'sel',0,'rst_all',false,'use_rst_all',false,'cinused',false,'ninstr',1}  hide_port_list={'c'}  block_type=mcode
      settings: xl_area=[0, 0, 0, 0, 0, 0, 0]  block_version=9.1
  xlreinterpretdsp48macro : xbsIndex_r4/MCode  mfname=xlreinterpretdsp48macro  explicit_period=off  period=1  dbl_ovrd=off  enable_stdout=off  enable_debug=off  suppress_output=off  defparams={'full',precision,'n_bits',n_bits,'bin_pt',bin_pt,'arith_type',arith_type}  hide_port_list={}  block_type=mcode
      settings: xl_area=[0, 0, 0, 0, 0, 0, 0]  block_version=9.1
  P : Outport  OutDataType=sfix(16)  OutScaling=2^0
  wires:
  xlreinterpretdsp48macro/1 -> P/1
  DSP48/1 -> xlreinterpretdsp48macro/1
  xlmacroissueengine/7 -> xlreinterpretdsp48macro/2
  xlmacroissueengine/6 -> DSP48/6
  xlmacroissueengine/5 -> DSP48/5
  xlmacroissueengine/4 -> DSP48/4
  xlmacroissueengine/3 -> DSP48/3
  xlmacroissueengine/2 -> DSP48/2
  xlmacroissueengine/1 -> DSP48/1
  b/1 -> xlmacroissueengine/2
  a/1 -> xlmacroissueengine/1

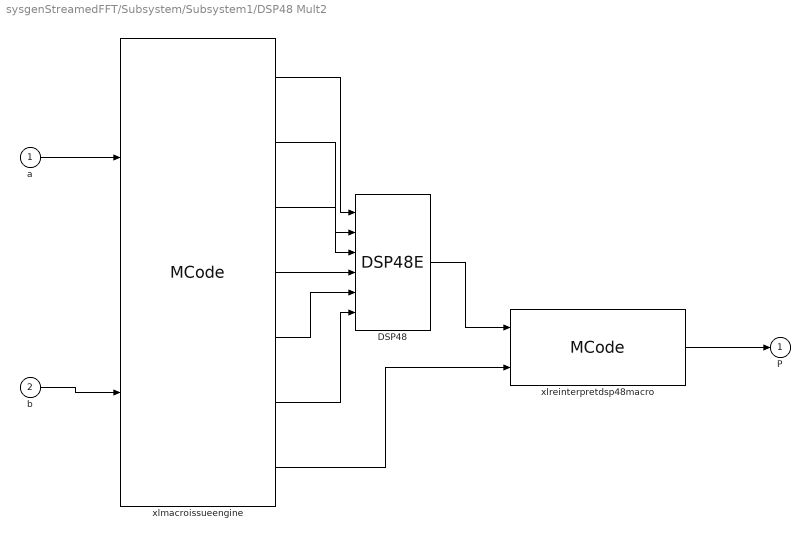
== system sysgenStreamedFFT/Subsystem/Subsystem1/DSP48 Mult2 ==
  a : Inport  OutDataType=sfix(16)  OutScaling=2^0
  b : Inport  Port=2  OutDataType=sfix(16)  OutScaling=2^0
  DSP48 : xbsIndex_r4/DSP48E  use_a=Direct from A Port  use_b=Direct from B Port  pattern_from_creg=off  pattern='000000000000'  mask_from_creg=off  pattern_mask='000000000000'  reset_preg=off  sel_rounding_mask=Select mask  use_op=off  use_creg=off  rst_all=off  en_all=off  use_pcin=off  use_carrycascin=off  use_multsignin=off  use_carryout=off  use_patterndetect=off  use_patternbdetect=off  use_overflow=off  use_underflow=off  use_acout=off  use_bcout=off  use_pcout=off  use_multsignout=off  use_carrycascout=off  pipeline_a=1  pipeline_b=1  pipeline_acout=1  pipeline_bcout=1  pipeline_c=off  pipeline_p=on  pipeline_mult=on  pipeline_opmode=on  pipeline_alumode=on  pipeline_carryin=on  pipeline_carryinsel=on  rst_a=off  rst_b=off  rst_c=off  rst_mult=off  rst_p=off  rst_carry_in=off  rst_alumode=off  rst_ctrl=off  en_a1=off  en_a2=off  en_b1=off  en_b2=off  en_c=off  en_mult=off  en_p=off  en_carry_in=off  en_alumode=off  en_multcarryin=off  en_ctrl=off  use_synth_model=off  addsub_mode=ONE48  xl_useadderonly=off  block_type=dsp48e
      settings: block_version=11.3
  xlmacroissueengine : xbsIndex_r4/MCode  mfname=xlissue_engine_v5  explicit_period=off  period=inf  dbl_ovrd=off  enable_stdout=off  enable_debug=off  suppress_output=on  defparams={'id_a1', 0,'id_a2', 0,'id_a3', 0,'id_a4', 0,'id_a5', 0,'id_a6', 0,'id_a7', 0,'id_b1', 0,'id_b2', 0,'id_b3', 0,'id_b4', 0,'id_b5', 0,'id_b6', 0,'id_b7', 0,'id_c0', 0,'id_c1', 0,'id_c2', 0,'id_c3', 0,'id_c4', 0,'id_c5', 0,'id_c6', 0,'id_c7', 0,'op_const0',5,'op_const1', 0,'op_const2', 0,'op_const3', 0,'op_const4', 0,'op_const5', 0,'op_const6', 0,'op_const7', 0,'alumode_const0',0,'alumode_const1', 0,'alumode_const2', 0,'alumode_const3', 0,'alumode_const4', 0,'alumode_const5', 0,'alumode_const6', 0,'alumode_const7', 0,'carry_in_sel0',0,'carry_in_sel1', 0,'carry_in_sel2', 0,'carry_in_sel3', 0,'carry_in_sel4', 0,'carry_in_sel5', 0,'carry_in_sel6', 0,'carry_in_sel7', 0,'external_cin0', 0,'external_cin1', 0,'external_cin2', 0,'external_cin3', 0,'external_cin4', 0,'external_cin5', 0,'external_cin6', 0,'external_cin7', 0,'reg_a',0,'reg_b',0,'reg_c',0,'reg_op',0,'mode0', 1,'mode1', 0,'mode2', 0,'mode3', 0,'mode4', 0,'mode5', 0,'mode6', 0,'mode7', 0,'ce_all',true,'use_ce_all',false,'sel',0,'rst_all',false,'use_rst_all',false,'cinused',false,'ninstr',1}  hide_port_list={'c'}  block_type=mcode
      settings: xl_area=[0, 0, 0, 0, 0, 0, 0]  block_version=9.1
  xlreinterpretdsp48macro : xbsIndex_r4/MCode  mfname=xlreinterpretdsp48macro  explicit_period=off  period=1  dbl_ovrd=off  enable_stdout=off  enable_debug=off  suppress_output=off  defparams={'full',precision,'n_bits',n_bits,'bin_pt',bin_pt,'arith_type',arith_type}  hide_port_list={}  block_type=mcode
      settings: xl_area=[0, 0, 0, 0, 0, 0, 0]  block_version=9.1
  P : Outport  OutDataType=sfix(16)  OutScaling=2^0
  wires:
  xlreinterpretdsp48macro/1 -> P/1
  DSP48/1 -> xlreinterpretdsp48macro/1
  xlmacroissueengine/7 -> xlreinterpretdsp48macro/2
  xlmacroissueengine/6 -> DSP48/6
  xlmacroissueengine/5 -> DSP48/5
  xlmacroissueengine/4 -> DSP48/4
  xlmacroissueengine/3 -> DSP48/3
  xlmacroissueengine/2 -> DSP48/2
  xlmacroissueengine/1 -> DSP48/1
  b/1 -> xlmacroissueengine/2
  a/1 -> xlmacroissueengine/1

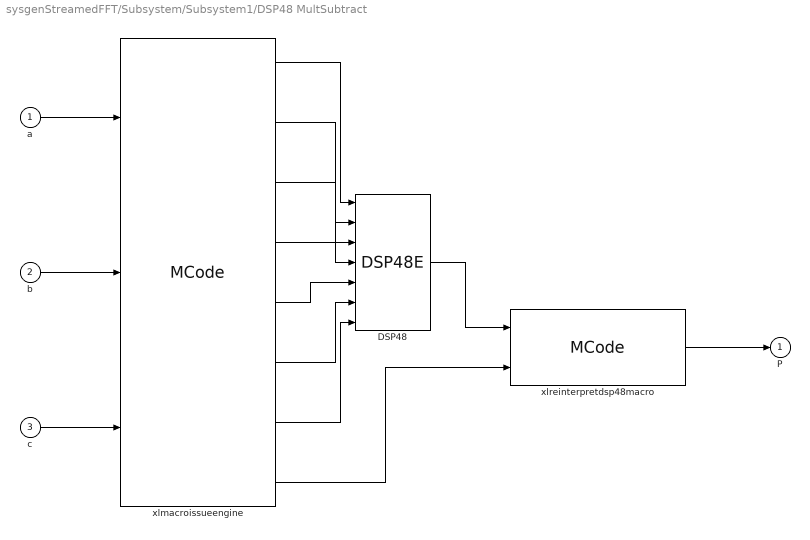
== system sysgenStreamedFFT/Subsystem/Subsystem1/DSP48 MultSubtract ==
  a : Inport  OutDataType=sfix(16)  OutScaling=2^0
  b : Inport  Port=2  OutDataType=sfix(16)  OutScaling=2^0
  c : Inport  Port=3  OutDataType=sfix(16)  OutScaling=2^0
  DSP48 : xbsIndex_r4/DSP48E  use_a=Direct from A Port  use_b=Direct from B Port  pattern_from_creg=off  pattern='000000000000'  mask_from_creg=off  pattern_mask='000000000000'  reset_preg=off  sel_rounding_mask=Select mask  use_op=off  use_creg=on  rst_all=off  en_all=off  use_pcin=off  use_carrycascin=off  use_multsignin=off  use_carryout=off  use_patterndetect=off  use_patternbdetect=off  use_overflow=off  use_underflow=off  use_acout=off  use_bcout=off  use_pcout=off  use_multsignout=off  use_carrycascout=off  pipeline_a=1  pipeline_b=1  pipeline_acout=1  pipeline_bcout=1  pipeline_c=on  pipeline_p=on  pipeline_mult=on  pipeline_opmode=on  pipeline_alumode=on  pipeline_carryin=on  pipeline_carryinsel=on  rst_a=off  rst_b=off  rst_c=off  rst_mult=off  rst_p=off  rst_carry_in=off  rst_alumode=off  rst_ctrl=off  en_a1=off  en_a2=off  en_b1=off  en_b2=off  en_c=off  en_mult=off  en_p=off  en_carry_in=off  en_alumode=off  en_multcarryin=off  en_ctrl=off  use_synth_model=off  addsub_mode=ONE48  xl_useadderonly=off  block_type=dsp48e
      settings: block_version=11.3
  xlmacroissueengine : xbsIndex_r4/MCode  mfname=xlissue_engine_v5  explicit_period=off  period=inf  dbl_ovrd=off  enable_stdout=off  enable_debug=off  suppress_output=on  defparams={'id_a1', 0,'id_a2', 0,'id_a3', 0,'id_a4', 0,'id_a5', 0,'id_a6', 0,'id_a7', 0,'id_b1', 0,'id_b2', 0,'id_b3', 0,'id_b4', 0,'id_b5', 0,'id_b6', 0,'id_b7', 0,'id_c1', 0,'id_c2', 0,'id_c3', 0,'id_c4', 0,'id_c5', 0,'id_c6', 0,'id_c7', 0,'op_const0',53,'op_const1', 0,'op_const2', 0,'op_const3', 0,'op_const4', 0,'op_const5', 0,'op_const6', 0,'op_const7', 0,'alumode_const0',3,'alumode_const1', 0,'alumode_const2', 0,'alumode_const3', 0,'alumode_const4', 0,'alumode_const5', 0,'alumode_const6', 0,'alumode_const7', 0,'carry_in_sel0',0,'carry_in_sel1', 0,'carry_in_sel2', 0,'carry_in_sel3', 0,'carry_in_sel4', 0,'carry_in_sel5', 0,'carry_in_sel6', 0,'carry_in_sel7', 0,'external_cin0', 0,'external_cin1', 0,'external_cin2', 0,'external_cin3', 0,'external_cin4', 0,'external_cin5', 0,'external_cin6', 0,'external_cin7', 0,'reg_a',0,'reg_b',0,'reg_c',0,'reg_op',0,'mode0', 1,'mode1', 0,'mode2', 0,'mode3', 0,'mode4', 0,'mode5', 0,'mode6', 0,'mode7', 0,'ce_all',true,'use_ce_all',false,'sel',0,'rst_all',false,'use_rst_all',false,'cinused',false,'ninstr',1}  hide_port_list={}  block_type=mcode
      settings: xl_area=[0, 0, 0, 0, 0, 0, 0]  block_version=9.1
  xlreinterpretdsp48macro : xbsIndex_r4/MCode  mfname=xlreinterpretdsp48macro  explicit_period=off  period=1  dbl_ovrd=off  enable_stdout=off  enable_debug=off  suppress_output=off  defparams={'full',precision,'n_bits',n_bits,'bin_pt',bin_pt,'arith_type',arith_type}  hide_port_list={}  block_type=mcode
      settings: xl_area=[0, 0, 0, 0, 0, 0, 0]  block_version=9.1
  P : Outport  OutDataType=sfix(16)  OutScaling=2^0
  wires:
  xlreinterpretdsp48macro/1 -> P/1
  DSP48/1 -> xlreinterpretdsp48macro/1
  xlmacroissueengine/8 -> xlreinterpretdsp48macro/2
  xlmacroissueengine/7 -> DSP48/7
  xlmacroissueengine/6 -> DSP48/6
  xlmacroissueengine/5 -> DSP48/5
  xlmacroissueengine/4 -> DSP48/4
  xlmacroissueengine/3 -> DSP48/3
  xlmacroissueengine/2 -> DSP48/2
  xlmacroissueengine/1 -> DSP48/1
  c/1 -> xlmacroissueengine/3
  b/1 -> xlmacroissueengine/2
  a/1 -> xlmacroissueengine/1
